simulink model "gm_combinedTxRx_ExternalMode"  (R2017b)
settings: Solver=FixedStepDiscrete  StartTime=0.0  StopTime=10.0  RelTol=1e-3
InitFcn:
  | modelSettings
undefined symbols (not defined in the file or in its folder): coeff, filt, j, RadioSampleRate, VibertiTracebackLength, xPreambleSeq
libraries: simulink x20, dsphdlfiltering x20, hdlsllib x10, hdlmdlgenlib x6, dspsigops x5, commseqgen3 x4, commdigbbndpm3 x3, commcrc2 x2, commcnvcod2 x2, commsource2 x1, dspstat3 x1, dspmlti4 x1
(part 5 of 5)

== system gm_combinedTxRx_ExternalMode/Combined TX and RX/Receiver HDL/Frame Recover/Gardner Timing Recovery/Gardner TED Blocks/Real Error/TED Buffer Update1 ==
  new data : Inport  SampleTime=1e-06
  strobe sum : Inport  Port=2  SampleTime=1e-06
  Enable_out2 : Inport  Port=3  OutDataTypeStr=boolean  SampleTime=1e-06
  Delay : Subsystem
      settings: MinAlgLoopOccurrences=on
  Delay1 : Subsystem
      settings: MinAlgLoopOccurrences=on
  Delay2 : Subsystem
      settings: MinAlgLoopOccurrences=on
  Delay3 : Subsystem
      settings: MinAlgLoopOccurrences=on
  Multiport Switch{,1..3} (4 alike) : MultiPortSwitch  DataPortOrder=Zero-based contiguous  DiagnosticForDefault=None  OutDataTypeStr=fixdt(1, 16, 10)  SampleTime=1e-06
  Zero bit : Constant  Value=fi(0,1,16,13,'hex','0000')  OutDataTypeStr=fixdt(1, 16, 13)  SampleTime=-1
  Middle Indx : Outport  InitialOutput=0
  oldest : Outport  Port=2  InitialOutput=0
  wires:
  new data/1 -> Multiport Switch3/4, Multiport Switch3/3
  strobe sum/1 -> Multiport Switch3/1, Multiport Switch2/1, Multiport Switch1/1, Multiport Switch/1
  Delay/1(out0) -> Multiport Switch/2
  Delay1/1(out0) -> Multiport Switch1/2, Multiport Switch/3
  Delay2/1(out0) -> Multiport Switch2/2, Multiport Switch1/3, Multiport Switch/4
  Delay3/1(out0) -> Multiport Switch3/2, Multiport Switch2/3, Multiport Switch1/4
  Multiport Switch/1 -> Delay/1(in0), oldest/1
  Multiport Switch1/1 -> Delay1/1(in0)
  Multiport Switch2/1 -> Delay2/1(in0), Middle Indx/1
  Multiport Switch3/1 -> Delay3/1(in0)
  Zero bit/1 -> Multiport Switch2/4
  Enable_out2/1 -> Delay3/Enable, Delay2/Enable, Delay1/Enable, Delay/Enable

== system gm_combinedTxRx_ExternalMode/Combined TX and RX/Receiver HDL/Frame Recover/Equalization and Demodulation/DFE/DFE/Map Symbol/Decision Directed ==
  eqOut : Inport  OutDataTypeStr=fixdt(1,16,14)  SampleTime=1e-06
  Compare To Zero : simulink/Logic and Bit Operations/Compare To Constant  relop=>=  const=hex2num('0000000000000000')  OutDataTypeStr=boolean
  Compare To Zero1 : simulink/Logic and Bit Operations/Compare To Constant  relop=>=  const=hex2num('0000000000000000')  OutDataTypeStr=boolean
  Complex to Real-Imag : ComplexToRealImag  SampleTime=1e-06
  QPSK Decisions : LookupNDDirect  Table="reshape([complex(-0.7071, -0.7071) complex(0.7071, -0.7071) complex(-0.7071, 0.7071) complex(0.7071, 0.7071)].', [2  2])"  DiagnosticForOutOfRangeInput=Error  SampleTime=1e-06  TableDataTypeStr=fixdt(1,16,15)
  decision : Outport  InitialOutput=0
  wires:
  eqOut/1 -> Complex to Real-Imag/1
  Compare To Zero/1 -> QPSK Decisions/1
  Compare To Zero1/1 -> QPSK Decisions/2
  Complex to Real-Imag/1 -> Compare To Zero/1
  Complex to Real-Imag/2 -> Compare To Zero1/1
  QPSK Decisions/1 -> decision/1

== system gm_combinedTxRx_ExternalMode/Combined TX and RX/Receiver HDL/Frame Recover/Equalization and Demodulation/DFE/DFE/Map Symbol/Delay ==
  in0 : Inport  OutDataTypeStr=fixdt(1, 16, 15)  SampleTime=1e-06
      settings: SignalType=complex
  Enable_out4 : EnablePort  OutDataTypeStr=boolean
  Delay : Delay  DelayLength=hex2num('3ff0000000000000')  InitialCondition=0  InputProcessing=Inherited
  out0 : Outport  OutDataTypeStr=fixdt(1, 16, 15)  InitialOutput=0
      settings: SignalType=complex
  wires:
  Delay/1 -> out0/1
  in0/1 -> Delay/1

== system gm_combinedTxRx_ExternalMode/Combined TX and RX/Receiver HDL/Frame Recover/Equalization and Demodulation/DFE/DFE/Map Symbol/HDL Counter ==
  in0 : Inport  OutDataTypeStr=boolean  SampleTime=1e-06
  Enable_out4 : EnablePort  OutDataTypeStr=boolean
  HDL Counter : hdlsllib/Sources/HDL Counter  CountType=Count limited  CountInit=hex2num('0000000000000000')  CountStep=hex2num('3ff0000000000000')  CountMax=hex2num('4110000000000000')  CountFromType=Initial value  CountFrom=hex2num('0000000000000000')  CountResetPort=on  CountLoadPort=off  CountEnbPort=off  CountDirPort=off  CountDataType=Unsigned  CountWordLen=32  CountFracLen=0  CountSampTime=1e-06
      settings: SourceProductBaseCode=HD
  out0 : Outport  OutDataTypeStr=uint32  InitialOutput=0
  wires:
  HDL Counter/1 -> out0/1
  in0/1 -> HDL Counter/1

== system gm_combinedTxRx_ExternalMode/Combined TX and RX/Receiver HDL/Frame Recover/Gardner Timing Recovery/Gardner TED Blocks/Imag Error/TED Buffer Update1/Delay ==
  in0 : Inport  OutDataTypeStr=fixdt(1, 16, 10)  SampleTime=1e-06
  Enable_out2 : EnablePort  OutDataTypeStr=boolean
  Delay : Delay  DelayLength=hex2num('3ff0000000000000')  InitialCondition=0  InputProcessing=Inherited
  out0 : Outport  OutDataTypeStr=fixdt(1, 16, 10)  InitialOutput=0
  wires:
  Delay/1 -> out0/1
  in0/1 -> Delay/1

== system gm_combinedTxRx_ExternalMode/Combined TX and RX/Receiver HDL/Frame Recover/Gardner Timing Recovery/Gardner TED Blocks/Imag Error/TED Buffer Update1/Delay1 ==
  in0 : Inport  OutDataTypeStr=fixdt(1, 16, 10)  SampleTime=1e-06
  Enable_out2 : EnablePort  OutDataTypeStr=boolean
  Delay1 : Delay  DelayLength=hex2num('3ff0000000000000')  InitialCondition=0  InputProcessing=Inherited
  out0 : Outport  OutDataTypeStr=fixdt(1, 16, 10)  InitialOutput=0
  wires:
  Delay1/1 -> out0/1
  in0/1 -> Delay1/1

== system gm_combinedTxRx_ExternalMode/Combined TX and RX/Receiver HDL/Frame Recover/Gardner Timing Recovery/Gardner TED Blocks/Imag Error/TED Buffer Update1/Delay2 ==
  in0 : Inport  OutDataTypeStr=fixdt(1, 16, 10)  SampleTime=1e-06
  Enable_out2 : EnablePort  OutDataTypeStr=boolean
  Delay2 : Delay  DelayLength=hex2num('3ff0000000000000')  InitialCondition=0  InputProcessing=Inherited
  out0 : Outport  OutDataTypeStr=fixdt(1, 16, 10)  InitialOutput=0
  wires:
  Delay2/1 -> out0/1
  in0/1 -> Delay2/1

== system gm_combinedTxRx_ExternalMode/Combined TX and RX/Receiver HDL/Frame Recover/Gardner Timing Recovery/Gardner TED Blocks/Imag Error/TED Buffer Update1/Delay3 ==
  in0 : Inport  OutDataTypeStr=fixdt(1, 16, 10)  SampleTime=1e-06
  Enable_out2 : EnablePort  OutDataTypeStr=boolean
  Delay3 : Delay  DelayLength=hex2num('3ff0000000000000')  InitialCondition=0  InputProcessing=Inherited
  out0 : Outport  OutDataTypeStr=fixdt(1, 16, 10)  InitialOutput=0
  wires:
  Delay3/1 -> out0/1
  in0/1 -> Delay3/1

== system gm_combinedTxRx_ExternalMode/Combined TX and RX/Receiver HDL/Frame Recover/Gardner Timing Recovery/Gardner TED Blocks/Real Error/TED Buffer Update1/Delay ==
  in0 : Inport  OutDataTypeStr=fixdt(1, 16, 10)  SampleTime=1e-06
  Enable_out2 : EnablePort  OutDataTypeStr=boolean
  Delay : Delay  DelayLength=hex2num('3ff0000000000000')  InitialCondition=0  InputProcessing=Inherited
  out0 : Outport  OutDataTypeStr=fixdt(1, 16, 10)  InitialOutput=0
  wires:
  Delay/1 -> out0/1
  in0/1 -> Delay/1

== system gm_combinedTxRx_ExternalMode/Combined TX and RX/Receiver HDL/Frame Recover/Gardner Timing Recovery/Gardner TED Blocks/Real Error/TED Buffer Update1/Delay1 ==
  in0 : Inport  OutDataTypeStr=fixdt(1, 16, 10)  SampleTime=1e-06
  Enable_out2 : EnablePort  OutDataTypeStr=boolean
  Delay1 : Delay  DelayLength=hex2num('3ff0000000000000')  InitialCondition=0  InputProcessing=Inherited
  out0 : Outport  OutDataTypeStr=fixdt(1, 16, 10)  InitialOutput=0
  wires:
  Delay1/1 -> out0/1
  in0/1 -> Delay1/1

== system gm_combinedTxRx_ExternalMode/Combined TX and RX/Receiver HDL/Frame Recover/Gardner Timing Recovery/Gardner TED Blocks/Real Error/TED Buffer Update1/Delay2 ==
  in0 : Inport  OutDataTypeStr=fixdt(1, 16, 10)  SampleTime=1e-06
  Enable_out2 : EnablePort  OutDataTypeStr=boolean
  Delay2 : Delay  DelayLength=hex2num('3ff0000000000000')  InitialCondition=0  InputProcessing=Inherited
  out0 : Outport  OutDataTypeStr=fixdt(1, 16, 10)  InitialOutput=0
  wires:
  Delay2/1 -> out0/1
  in0/1 -> Delay2/1

== system gm_combinedTxRx_ExternalMode/Combined TX and RX/Receiver HDL/Frame Recover/Gardner Timing Recovery/Gardner TED Blocks/Real Error/TED Buffer Update1/Delay3 ==
  in0 : Inport  OutDataTypeStr=fixdt(1, 16, 10)  SampleTime=1e-06
  Enable_out2 : EnablePort  OutDataTypeStr=boolean
  Delay3 : Delay  DelayLength=hex2num('3ff0000000000000')  InitialCondition=0  InputProcessing=Inherited
  out0 : Outport  OutDataTypeStr=fixdt(1, 16, 10)  InitialOutput=0
  wires:
  Delay3/1 -> out0/1
  in0/1 -> Delay3/1

== matlab function gm_combinedTxRx_ExternalMode/Combined TX and RX/Receiver HDL/Frame Recover/Frequency Recovery/Lock Detector/MATLAB Function/RxTxFixedPointLibrary_c1_MATLAB_Function ==
  data: u input; y output
function y = abs(u)

y = fi(u,0,16,10);

== matlab function gm_combinedTxRx_ExternalMode/Combined TX and RX/Receiver HDL/Viterbi Decode/Buffer/MATLAB Function1/RxTxFixedPointLibrary_c2_MATLAB_Function1 ==
  data: packetLen input; valid input; enablePop output; validOut output; crcStart input; viterbiReset output; crcOut output
function [enablePop,validOut,viterbiReset,crcOut] = manageCurrentDequeue(packetLen, valid, crcStart)

persistent currentBitsInBuffer

bitsPerCycle = uint16(2);
%bitsPerCycleDouble = uint16(4);
viterbiTracebackLengthDouble = uint16(34*2) + uint16(0);

if isempty(currentBitsInBuffer)
    currentBitsInBuffer = uint16(0);
end

if currentBitsInBuffer > viterbiTracebackLengthDouble
    currentBitsInBuffer = currentBitsInBuffer - bitsPerCycle;
    enablePop = true;
    viterbiReset = false;
    crcOut = false;
    validOut = true;
% Trigger packet at length of packet data and let Viterbi eat remaining
% data needed for traceback
elseif currentBitsInBuffer == viterbiTracebackLengthDouble
    currentBitsInBuffer = currentBitsInBuffer - bitsPerCycle;
    enablePop = true;
    viterbiReset = false;
    crcOut = true;
    validOut = false;
% Flush remaining buffered data
elseif (currentBitsInBuffer < viterbiTracebackLengthDouble) &&...
       (currentBitsInBuffer > uint16(0))
    currentBitsInBuffer = currentBitsInBuffer - bitsPerCycle;
    enablePop = true;
    viterbiReset = false;
    crcOut = false;
    validOut = false;
else
    if valid
        if crcStart
            currentBitsInBuffer = packetLen + viterbiTracebackLengthDouble + uint16(0);%bitsPerCycleDouble;
            enablePop = true;
            viterbiReset = true;
            crcOut = false;
            validOut = true;
        else
            enablePop = false;
            viterbiReset = false;
            crcOut = false;
            validOut = false;
        end
    else
        enablePop = false;
        viterbiReset = false;
        crcOut = false;     
        validOut = false;
    end
end

== matlab function gm_combinedTxRx_ExternalMode/Combined TX and RX/DMA Model Driver/DMA Model Driver ==
  data: driver input; payload output; valid output boolean; enable input
function [payload,valid] = fcn(driver, enable)
%#codegen

persistent indx mode pSize

if isempty(indx)
    pSize = fi(200,0,64,0); % Size in bytes (Must be multiple of 32 bits) cannot exceed uint16 max
    indx = pSize;
    mode = int8(0);
end

setting = uint16(25*8);

if enable && driver
    valid = true;
    switch mode
        case int8(0) % Fresh packet start
            if setting>0
                pSize = fi(setting,0,64,0);
                payload = fi(setting,0,64,0);%Upper bits
                mode = int8(1);
                indx = fi(0,0,64,0);
                %fprintf('(TX) Sending new packet with length: %u\n',uint64(pSize));
            else
                valid = false;
                payload = fi(0,0,64,0);
            end
        otherwise
            indx = fi(indx + fi(8,0,64,0),0,64,0);
            if indx == fi(8,0,64,0)
               payload = fi(0,0,64,0);
               payload = bitset(payload,1,1);
            elseif indx == pSize
                payload = fi(uint64(18446744073709551615),0,64,0); % All ones
          else
                payload = fi(uint64(12297829382473034410),0,64,0);%sum(2.^[0:2:14])); % Alternating ones and zeros
            end
            if indx == pSize % reached end of frame
                mode = int8(0);
            end
    end
else
    valid = false;
    payload = fi(0,0,64,0);
end

== matlab function gm_combinedTxRx_ExternalMode/Combined TX and RX/Transmitter HDL/Packet Generation/Payload/MATLAB Function/RxTxFixedPointLibrary_c4_MATLAB_Function ==
  data: enable input; reset output; mode output
function [reset,mode] = fcn(enable)

persistent counter

if isempty(counter)
   counter = uint8(0);
end

if enable
    counter = uint8(34*2); % tracebacklength*2
    mode = uint8(1);
    reset = true;
elseif counter>uint8(0)
    counter = counter - 1;
    mode = uint8(1);
    reset = false;
else
    mode = uint8(0);
    reset = false;
end

== matlab function gm_combinedTxRx_ExternalMode/Combined TX and RX/Receiver HDL/Frame Recover/Gardner Timing Recovery/TED Lock Detector/MATLAB Function/RxTxFixedPointLibrary_c5_MATLAB_Function ==
  data: u input; y output
function y = abs(u)

y = fi(u,0,16,15);

== matlab function gm_combinedTxRx_ExternalMode/Combined TX and RX/Transmitter HDL/Packet Generation/Payload/Subsystem/MATLAB Function3/RxTxFixedPointLibrary_c9_MATLAB_Function3 ==
  data: start input; enable output; done input
function enable = latch(start,done)

persistent state

if isempty(state)
   state = false; 
end

if start
    enable = true;
    state = true;
elseif done
    enable = true;
    state = false;
else
    enable = state;
end

== matlab function gm_combinedTxRx_ExternalMode/Combined TX and RX/Receiver HDL/Frame Recover/Equalization and Demodulation/2 Bit Descrambler/MATLAB Function/MATLAB Function/RxTxFixedPointLibrary_c10_MATLAB_Function ==
  data: bits input; bufferA output; reset input; bufferB output
function [bufferA, bufferB] = BufferSelect(bits,reset)

persistent buffer

% Constants
initBuffer = logical([0 1 0 0 0 1 0]);

% Async
if isempty(buffer)
    buffer = initBuffer;
end

% Reset/Sync
if reset
    bufferA = initBuffer;
    bufferB = [bits(1),initBuffer(1:end-1)];
    buffer = [bits(2),bits(1),initBuffer(1:end-2)];
else
    bufferA = buffer;
    bufferB = [bits(1),buffer(1:end-1)];
    buffer = [bits(2),bits(1),buffer(1:end-2)];    
end

== matlab function gm_combinedTxRx_ExternalMode/Combined TX and RX/Receiver HDL/CRC Check and DMA Pack/DMA Interface/Bit Packer/RxTxFixedPointLibrary_c11_Bit_Packer ==
  data: bitIn input; byteOut output; startIn input; endIn input; err input; validIn input; validOut output; startOut output
function [byteOut,validOut,startOut] = BitPacker(bitIn, startIn, endIn, err, validIn)

% This block will pack bits into bytes with start boundaries


% Constants
bits2Pack = uint8(64); % byteReg must contain this many bits
zero64 = fi(0,0,64,0);
% NOTE: Frames but be a multiple of bits2Pack or bits will be trimmed from
% end

persistent byteReg byteIndx setStartFlag

if isempty(byteIndx)
    byteReg  = fi(0,0,64,0);
    byteIndx = uint8(1);
    setStartFlag = false;
end

if validIn
    if startIn % Reset
        byteReg = bitset(zero64,1,bitIn);
        byteIndx = uint8(2);
        validOut = false;
        setStartFlag = true;
        startOut = false;
    else
        byteReg = bitset(byteReg,byteIndx,bitIn);
        if byteIndx >= bits2Pack
            byteIndx = uint8(1);
            validOut = true;
            startOut = setStartFlag;
            setStartFlag = false;
        else
            byteIndx = byteIndx + uint8(1);
            validOut = false;
            startOut = false;
        end
    end
elseif endIn % Append error bit to last byte
    byteReg = fi(err,0,64,0);
    validOut = true;
    startOut = false;
else
    validOut = false;
    startOut = false;
end

byteOut = byteReg;

== matlab function gm_combinedTxRx_ExternalMode/Combined TX and RX/Receiver HDL/Frame Recover/Enable Equalizer and Packet Decode (Latch)/RxTxFixedPointLibrary_c12_Enable_Equalizer_and_Packet_Decode__L ==
  data: start input; enable output; validIn input
function enable = Counter(start,validIn)

persistent count maxCount lastEOF

if isempty(count)
    count = uint32(0);
    maxCount = uint32(2^16); % Largest possible packet length
    lastEOF = false;
end

eof = false;

if validIn
    % Got a barker preamble start allowing data into equalizer
    if start
        count = maxCount;
    end
    
    % Check on change from true to false
    if lastEOF && ~eof
        %     fprintf('Frame end reached\n');
        count = uint32(0);
    end
    lastEOF = eof;
    
    % Past end of max frame size
    if count>0
        count = count - uint32(1);
    end
    
    % Enable downstream
    enable = count>uint32(0);
else
    enable = false;
end

== matlab function gm_combinedTxRx_ExternalMode/Combined TX and RX/Receiver HDL/Frame Recover/Equalization and Demodulation/Header Controller/Header Controller/RxTxFixedPointLibrary_c15_Header_Controller ==
  data: enableDownstream output; headerStart input; packetLenBitsOut output; data input; resetViterbi output; crcStart output; status output; s1 output; s2 output
function [enableDownstream,packetLenBitsOut,resetViterbi,crcStart,status,s1,s2] = EvalHeader(headerStart, data)

persistent counter sum1 sum2 packetLenBits lastMode savedPacketLenBits

% The header contains 16 bits, but each bit is duplicated to make checking
% easier
%
% Note this block works on symbols (2bits) but 1 symbol -> 1 decoded bit
%
% PacketLength = (Data+CRC+40(TB)+68)/CodeRate
%
% NOTE TAIL BITS HERE ARE REALLY USED TO DEAL WITH VITERBI LAG SO:
% TailBitsWithLagPadding > TracebackLength

%% Constants
numHeaderBits = uint8(16); % Header is this many bits
powersOfTwo = uint32([1 2 4 8 16 32 64 128 256 512 1024 2048 4096 8192 16384 32768]);
CodeRateINV = uint32(2);%1/CodeRate;
TailBitsWithLagPadding = uint32(uint32(40)+34*2+1); % was +1
% Flag when CRC porition of packet starts relative to header
crcSignalStartLocation = uint32((TailBitsWithLagPadding)*CodeRateINV); % Must be even

% Async
if isempty(counter)
    packetLenBits = uint32(0);
    sum1 = uint32(0);
    sum2 = uint32(0);
    counter = uint8(numHeaderBits);
    lastMode = uint8(3);
    savedPacketLenBits = uint16(0);
end


%% Sync
% Got a header now enable certain mode
if headerStart
    mode = uint8(0);
else
    mode = lastMode;
end

switch mode
    %% Reset on preamble flag and setup for header processing
    case uint8(0)
        crcStart = false;
        resetViterbi = false;
        enableDownstream = false;
        sum1 = uint32(0);
        sum2 = uint32(0);
        counter = uint8(1);
        lastMode = uint8(1); % Go to next state
        packetLenBitsOut = uint16(0);
        status = uint8(0); s1 = uint32(0); s2 = uint32(0);
        
    %% Process header
    case 1 
        crcStart = false;
        enableDownstream = false;
        
        % Convert header bits (bit by bit)
        if data(1)
            sum1 = sum1 + powersOfTwo(counter);
        end
        if data(2)
            sum2 = sum2 + powersOfTwo(counter);
        end
        counter = counter + uint8(1);
        
        if counter>numHeaderBits
            % Check header
            if sum1~=sum2 % Fail
                packetLenBits = uint32(0);
                lastMode = uint8(3);
                resetViterbi = false;
                packetLenBitsOut = uint16(0);
                savedPacketLenBits = uint16(0);
                status = uint8(2); s1 = sum1; s2 = sum2;
            else % Pass
                % Saved header info and trigger downstream
                packetLenBits = uint32(sum1);
                lastMode = uint8(2);
                resetViterbi = true;
                packetLenBitsOut = uint16(sum1-crcSignalStartLocation);
                savedPacketLenBits = uint16(sum1-crcSignalStartLocation);
                status = uint8(1); s1 = sum1; s2 = sum2;
            end
        else
            status = uint8(0); s1 = uint32(0); s2 = uint32(0);
            packetLenBitsOut = uint16(0);
            resetViterbi = false;
        end
        
    %% Decrement sample counter
    case 2 
        status = uint8(0); s1 = uint32(0); s2 = uint32(0);
        resetViterbi = false;
        crcStart = (packetLenBits==crcSignalStartLocation);
        if packetLenBits>uint32(0)
            enableDownstream = true;
            packetLenBits = packetLenBits - uint32(2); % We get 2 bits each call
            packetLenBitsOut = savedPacketLenBits;
        else
            enableDownstream = false;
            lastMode = uint8(3);
            packetLenBitsOut = uint16(0); %Reset
            savedPacketLenBits = uint16(0);%Reset
        end
            
    %% Not processing anything
    otherwise % mode>2
        status = uint8(0); s1 = uint32(0); s2 = uint32(0);
        crcStart = false;
        resetViterbi = false;
        enableDownstream = false;
        packetLenBitsOut = uint16(0);
end

== matlab function gm_combinedTxRx_ExternalMode/Combined TX and RX/Receiver HDL/Frame Recover/Frequency Recovery/PED/RxTxFixedPointLibrary_c16_PED ==
  data: In input; e output
function e  = PED(In)

OP2 = real(In);
OP1 = imag(In);

Real = OP2;
Imag = OP1;

if (bitget(Real,16)==true) % real component is negative
    OP1 = fi(-Imag,1,16,13);
end
if (bitget(Imag,16)==true) % imaginary component is negative
    OP2 = fi(-Real,1,16,13);
end

e= fi(OP1-OP2,1,16,10);

%e = sign(real(In)).*imag(In) - sign(imag(In)).*real(In);

== matlab function gm_combinedTxRx_ExternalMode/Combined TX and RX/Transmitter HDL/DMA Interface/DMA Control/RxTxFixedPointLibrary_c18_DMA_Control ==
  data: byteIn input; bitOut output; validIn input; validOut output; startOut output; payloadLength output; readyForInput output; EOF input
function [bitOut,validOut,startOut,payloadLength,readyForInput] = DMA_Control(byteIn,validIn,EOF)

% This block converts the byte input pipeline into bits and extract the
% length the packet into its own signal

persistent wordBuffer bitCounter payloadLenBuff mode inputByteCounter

bitsInInput = uint8(64);
bytesInInput = uint16(8);

if isempty(wordBuffer)
    wordBuffer = fi(0,0,64,0); % Must match number of bits defined by bitsInInput
    bitCounter = uint8(0);
    payloadLenBuff = uint16(0);
    mode = uint8(0);
    inputByteCounter = uint16(0);
end

%% Payload length setup
% Capture first payload length byte(s)
if validIn && (mode == uint8(0))
    mode = uint8(2);
    payloadLenBuff = uint16(byteIn);
    % Set outputs
    bitOut = false;
    validOut = false;
    startOut = true;
    payloadLength = uint16(0);
    readyForInput = true;
    % Reset counters
    inputByteCounter = bytesInInput;% Reset
    bitCounter = uint8(1);% Reset
    
%% Payload output
elseif (bitCounter > uint8(0))  && (mode==uint8(2))
    % Set outputs
    if bitCounter==uint8(1)
        bitOut = bitget(byteIn,1)>0;
        wordBuffer = byteIn; % Save byte
    else
        bitOut = bitget(wordBuffer,bitCounter)>0;
    end
    startOut = false;
    payloadLength = uint16(payloadLenBuff);
    validOut = true;
    % Set flag to DMA and next mode
    if bitCounter >= uint8(bitsInInput)
        bitCounter = uint8(1); % Reset
        % If we've processed all the bytes we need to wait for downstream
        % to be done
        if inputByteCounter<payloadLenBuff
            readyForInput = true; % Tell them we need next byte
            % Bytes processed
            inputByteCounter = inputByteCounter + bytesInInput;    
        else
            readyForInput = false; % Hold DMA off for now, next call will go to EOF
            mode = uint8(3);
        end
    else
        bitCounter = bitCounter+uint8(1);
        readyForInput = false;
    end
    
% Waiting for EOF from packet generation
elseif (mode==uint8(3))
    bitOut = false;
    validOut = true; % Keep downstream processing going
    startOut = false;
    payloadLength = uint16(payloadLenBuff);
    if EOF % Done with frame now ask for more data
        readyForInput = true;
        mode = uint8(0);% Reset
    else
        readyForInput = false;
    end
    
else % not-valid and need another byte
    bitOut = false;
    if mode == uint8(0)
        validOut = true; % Let LFSR Run
    else
        validOut = false;
    end
    startOut = false;
    payloadLength = uint16(0);
    readyForInput = true;
end

== matlab function gm_combinedTxRx_ExternalMode/Combined TX and RX/Transmitter HDL/Packet Generation/Payload/HDL Scrambler 2 bits/Buffer Manage/RxTxFixedPointLibrary_c20_Buffer_Manage ==
  data: bit1 input; bit2 input; outBuffer output; reset input
function outBuffer = fcn(bit1, bit2, reset)
%#codegen

init_buffer = logical([0 1 0 0 0 1 0]);

persistent buffer

if isempty(buffer)
    buffer = init_buffer;
end

if reset
    outBuffer = init_buffer;
    buffer = init_buffer;
    %outBuffer = [init_buffer(3:end),bit1,bit2];
    %buffer = [buffer(3:end),bit1,bit2];    
else
    outBuffer = [bit2,bit1,buffer(1:end-2)];
    buffer = [bit2,bit1,buffer(1:end-2)];
end

== matlab function gm_combinedTxRx_ExternalMode/Combined TX and RX/Transmitter HDL/Packet Generation/Tx Controller/RxTxFixedPointLibrary_c24_Tx_Controller ==
  data: modeOut output; headerData output; data output; payloadBit input; payloadSize input; count input; start input; dataStart output; dataEnd output; preambleReset output
function [modeOut, headerData, data, dataStart, dataEnd, preambleReset] = fcn(payloadBit,payloadSize,count, start)

% When we get a start flag buffers are reset and the next cycle with start
% in mode 0

% Reset: New payload size is passed at an int16
% 


persistent  headerBits numPayloadBits mode

numHeaderBits = uint32(16);
AGCBarkerSymbols = 160+28;
EQTrainingSymbols = 250; % 2 bits per symbol => 250 symbols
preambleBits = uint32(EQTrainingSymbols+AGCBarkerSymbols-0);
CRCLength = 32;
CRCGeneratorLag = CRCLength+2+0; % additional 1 is from reset of encoder
CodeRate = 2;
lagBits = 40+68;
viterbiTraceback = uint32(34*2);

% Async/Init
if isempty(numPayloadBits)
    % Sizes of frame sections
    numPayloadBits = uint32(0); 
    %headerBits = zeros(1,numHeaderBits)>0;
    headerBits = uint16(0);
    mode = uint8(4);
end

% Synchronous
switch mode
    case uint8(0) % Reset
        % Move to next mode on next input/clock
        mode = uint8(1);
        % Convert payloadSize to bits
        numPayloadBits = uint32(bitshift(payloadSize,3)+CRCLength);
        %headerBits = logical(bitget(CodeRate*(payloadSize+CRCLength),1:numHeaderBits));
        headerBits = uint16(bitshift((bitshift(payloadSize,3)+CRCLength+lagBits),1));        
        % Set outputs
        modeOut = uint8(4);
        headerData = false;
        data = false; % Not used downstream
        dataStart = false;
        dataEnd = false;
        preambleReset = true;
    case uint8(1) % Preamble
        % Set Next Mode
        if count>=(preambleBits)
            preambleReset = false;
            mode = uint8(2);
        elseif count==uint32(1)
            preambleReset = false;
            mode = uint8(1);
        else
            preambleReset = false;
            mode = uint8(1);
        end
        % Set outputs
        modeOut = uint8(1);
        headerData = false;
        % Start outputing data early to compensate for CRC lag
        if count>=(preambleBits+numHeaderBits-CRCGeneratorLag)
           data = payloadBit;
           % Set flag on first payload bit
           dataStart = count == (preambleBits+numHeaderBits-CRCGeneratorLag);
        else
           data = false;         
           dataStart = false;
        end
        dataEnd = false;
    case uint8(2) % Header bits
        % Set Next Mode
        if count>=(preambleBits+numHeaderBits)
            mode = uint8(3);
        else
            mode = uint8(2);
        end
        % Set outputs
        modeOut = uint8(2);
        %headerData = headerBits(count-preambleBits);
        headerData = bitget(headerBits,count-preambleBits)>0;
        data = payloadBit;
        dataStart = false;
        dataEnd = false;
        preambleReset = false;
    case uint8(3) % Payload bits and CRC
        % Set Next Mode
        if count>=(preambleBits+numHeaderBits+numPayloadBits+viterbiTraceback)%+CRCGeneratorLag)
            % Will coencide with last CRC Bit (NOT TRUE ANYMORE WILL BE ON
            % LAST TRACEBACK PADDING BIT)
            mode = uint8(4);
        else
            mode = uint8(3);
        end
        % Set outputs
        modeOut = uint8(3);        
        headerData = false;
        data = payloadBit;
        % Set flag on last payload bit
        dataStart = false;
        dataEnd =   ( count==(preambleBits+numHeaderBits+numPayloadBits-CRCLength-CRCGeneratorLag-1) );
        preambleReset = false;
    otherwise %case uint8(4) % Waiting for data
        % Chilling for new start
        if start
           mode = uint8(0); 
        else
           mode = uint8(4);
        end
        % Set outputs
        modeOut = uint8(4);
        headerData = false;
        data = false; % Not used downstream
        dataStart = false;
        dataEnd = false;
        preambleReset = false;
end

== matlab function gm_combinedTxRx_ExternalMode/Combined TX and RX/Receiver HDL/Viterbi Decode/Buffer/MATLAB Function/RxTxFixedPointLibrary_c26_MATLAB_Function ==
  data: valid input; enable output; start input; crcEnd input
function enable = latch(valid,start,crcEnd)

persistent state

if isempty(state)
    state = false;
end

if start
    enable = true && valid;
    state = true;
elseif crcEnd
    enable = true && valid;
    state = false;
else 
    enable = state && valid;
end
